simulink library "Radar_Block"  (R2018b)
settings: Solver=VariableStepAuto  StartTime=0.0  StopTime=10.0  RelTol=1e-3
undefined symbols (not defined in the file): ac1dyn_alt0_ft, ac1dyn_lat0_rad, ac1dyn_lon0_rad, uas_rdr_az_bias_rad, uas_rdr_az_random_stddev_rad, uas_rdr_az_tau_s, uas_rdr_debugMode, uas_rdr_dt_s, uas_rdr_el_bias_rad, uas_rdr_el_random_stddev_rad, uas_rdr_el_tau_s, uas_rdr_RCPR_Mode, uas_rdr_RCPR_Range_ft, uas_rdr_reported_errorCovRAE, uas_rdr_rng_bias_ft, uas_rdr_rng_random_stddev_ft, uas_rdr_rng_tau_s, uas_rdr_rngdot_bias_ftps, uas_rdr_rngdot_random_stddev_ftps, uas_rdr_rngdot_tau_s, uas_rdr_seed1, uas_rdr_seed2, uas_rdr_seed3, uas_rdr_seed4, uas_rdr_sns_for_azimuth_deg, uas_rdr_sns_for_elevation_deg
libraries: simulink x7, signalsLib x1, ExtractCovDiag x1
settings Model: Creator=RA24876  LastModifiedBy=BI28030
settings SFSimCC: SimUseLocalCustomCode=off
settings RTWCC: RTWUseLocalCustomCode=off
settings CodeAppCC: StateflowObjectComments=on

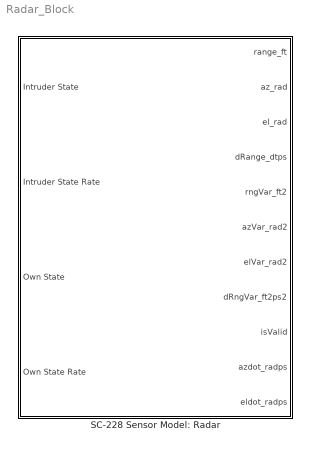
== system Radar_Block ==
  SC-228 Sensor Model: Radar : Subsystem  mask(Tracked Surveillance: Radar){dt_s=uas_rdr_dt_s, lat0_rad=ac1dyn_lat0_rad, lon0_rad=ac1dyn_lon0_rad, alt0_ft=ac1dyn_alt0_ft, sns_for_azimuth_deg=uas_rdr_sns_for_azimuth_deg, sns_for_elevation_deg=uas_rdr_sns_for_elevation_deg, debugMode=uas_rdr_debugMode, rng_random_stddev_ft=uas_rdr_rng_random_stddev_ft, rng_bias_ft=uas_rdr_rng_bias_ft, rng_tau_s=uas_rdr_rng_tau_s, seed1=uas_rdr_seed1, RCPR_Mode=uas_rdr_RCPR_Mode, RCPR_Range_ft=uas_rdr_RCPR_Range_ft, az_random_stddev_rad=uas_rdr_az_random_stddev_rad, az_bias_rad=uas_rdr_az_bias_rad, az_tau_s=uas_rdr_az_tau_s, seed2=uas_rdr_seed2, el_random_stddev_rad=uas_rdr_el_random_stddev_rad, el_bias_rad=uas_rdr_el_bias_rad, el_tau_s=uas_rdr_el_tau_s, seed3=uas_rdr_seed3, rngdot_random_stddev_ftps=uas_rdr_rngdot_random_stddev_ftps, rngdot_bias_ftps=uas_rdr_rngdot_bias_ftps, rngdot_tau_s=uas_rdr_rngdot_tau_s, seed4=uas_rdr_seed4, covRAE=uas_rdr_reported_errorCovRAE}
      mask prompts: dt_s "Timestep"; lat0_rad "ENU Origin Latitude"; lon0_rad "ENU Origin Longitude"; alt0_ft "ENU Origin Altitude"; sns_for_azimuth_deg "Field of Regard: Azimuth Limit (deg)"; sns_for_elevation_deg "Field of Regard: Elevation Limit (deg)"; debugMode "Whether to run in debug mode with inifinite detection range"; rng_random_stddev_ft "Range Random Error Standard Deviation"; rng_bias_ft "Range Bias"; rng_tau_s "Correlation Time"; seed1 "Random Seed"; RCPR_Mode "RCPR Mode (1 = minimum range enabled, 0 = not enabled)"; RCPR_Range_ft "RCPR Range (ft)"; az_random_stddev_rad "Azimuth Random Error Standard Deviation"; az_bias_rad "Azimuth Bias"; az_tau_s "Correlation Time"; seed2 "Random Seed"; el_random_stddev_rad "Elevation Random Error Standard Deviation"; el_bias_rad "Elevation Bias"; el_tau_s "Correlation Time"; seed3 "Random Seed"; rngdot_random_stddev_ftps "Range Rate Random Error Standard Deviation"; rngdot_bias_ftps "Range Rate Bias"; rngdot_tau_s "Correlation Time"; seed4 "Random Seed"; covRAE "Error Covariance"
      mask help: Additive noise model of an on-board radar
      mask Help:
      | Additive noise model of an on-board radar.  Independent noise is added to
      | each of range, azimuth, elevation and their rates.  Noise is colored using
      | weights determined by time constant parameters.
      | 
      | Output takes the form of a AircraftEstimate data bus and a 6x6 error covariance
      | matrix in North-East-Down.  State order in error covariance output is
      | [ posN posE posD velN velE velD ].
      mask DialogControl ParameterTabVar0 Prompt: Tab
      mask DialogControl ParameterTabVar01 Prompt: Range
      mask DialogControl ParameterTabVar012 Prompt: Azimuth
      mask DialogControl ParameterTabVar0123 Prompt: Elevation
      mask DialogControl ParameterTabVar01234 Prompt: Range rate
      mask DialogControl ParameterTabVar01234567 Prompt: Covariance

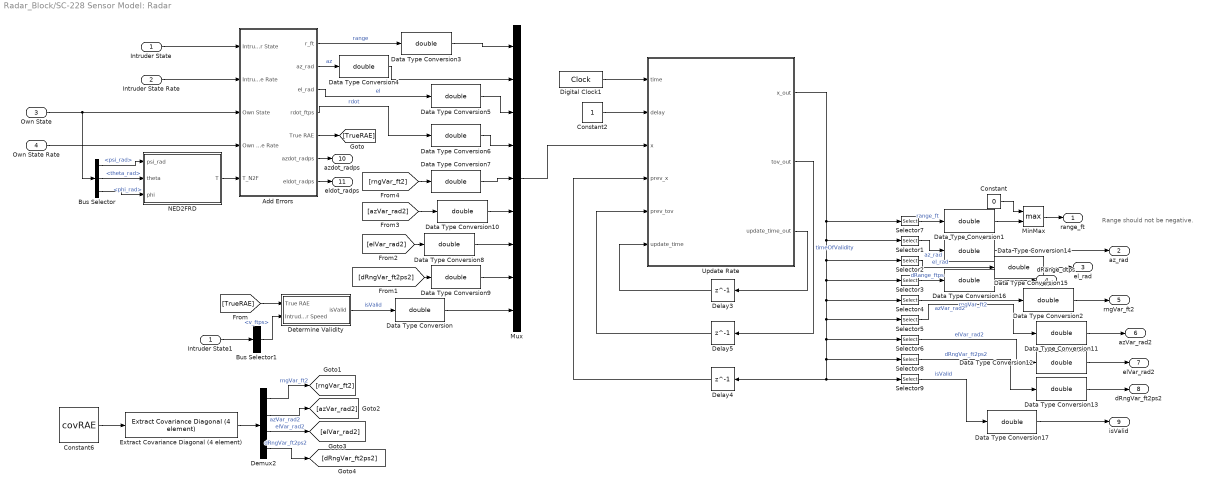
== system Radar_Block/SC-228 Sensor Model: Radar ==
  note: Range should not be negative.
  Intruder State : Inport  OutDataTypeStr=Bus: AircraftState
  Intruder State Rate : Inport  Port=2  OutDataTypeStr=Bus: AircraftStateRate
  Own State : Inport  Port=3  OutDataTypeStr=Bus: AircraftState
  Own State Rate : Inport  Port=4  OutDataTypeStr=Bus: AircraftStateRate
  Add Errors : Subsystem
  Bus Selector : BusSelector  OutputSignals=psi_rad,theta_rad,phi_rad
  Bus Selector1 : BusSelector  OutputSignals=v_ftps
  Constant : Constant  Value=0
  Constant2 : Constant
  Constant6 : Constant  Value=covRAE
  Data Type Conversion{,1..17} (18 alike) : DataTypeConversion  OutDataTypeStr=double
  Delay3 : Delay  DelayLength=1  InitialCondition=1
  Delay4 : Delay  DelayLength=1  InitialCondition=0
  Delay5 : Delay  DelayLength=1  InitialCondition=0
  Demux2 : Demux
  Determine Validity : Subsystem
  Digital Clock1 : DigitalClock  SampleTime=0.1
  Extract Covariance Diagonal (4 element) : ExtractCovDiag/Extract Covariance Diagonal (4 element)  SystemSampleTime=-1
  Intruder State1 : InportShadow  OutDataTypeStr=Bus: AircraftState
  MinMax : MinMax  Function=max  Inputs=2
  Mux : Mux  Inputs=9
  NED2FRD : MATLAB Function  TreatAsAtomicUnit=on
  Selector1 : Selector  InputPortWidth=9  IndexOptions=Index vector (dialog)  Indices=[2]  OutputSizes=1
  Selector2 : Selector  InputPortWidth=9  IndexOptions=Index vector (dialog)  Indices=[3]  OutputSizes=1
  Selector3 : Selector  InputPortWidth=9  IndexOptions=Index vector (dialog)  Indices=[4]  OutputSizes=1
  Selector4 : Selector  InputPortWidth=9  IndexOptions=Index vector (dialog)  Indices=[5]  OutputSizes=1
  Selector5 : Selector  InputPortWidth=9  IndexOptions=Index vector (dialog)  Indices=[6]  OutputSizes=1
  Selector6 : Selector  InputPortWidth=9  IndexOptions=Index vector (dialog)  Indices=[7]  OutputSizes=1
  Selector7 : Selector  InputPortWidth=9  IndexOptions=Index vector (dialog)  Indices=[1]  OutputSizes=1
  Selector8 : Selector  InputPortWidth=9  IndexOptions=Index vector (dialog)  Indices=[8]  OutputSizes=1
  Selector9 : Selector  InputPortWidth=9  IndexOptions=Index vector (dialog)  Indices=[9]  OutputSizes=1
  Update Rate : MATLAB Function  TreatAsAtomicUnit=on
  range_ft : Outport
  az_rad : Outport  Port=2
  el_rad : Outport  Port=3
  dRange_dtps : Outport  Port=4
  rngVar_ft2 : Outport  Port=5
  azVar_rad2 : Outport  Port=6
  elVar_rad2 : Outport  Port=7
  dRngVar_ft2ps2 : Outport  Port=8
  isValid : Outport  Port=9
  azdot_radps : Outport  Port=10
  eldot_radps : Outport  Port=11
  wires:
  Data Type Conversion13/1 -> dRngVar_ft2ps2/1
  Data Type Conversion12/1 -> elVar_rad2/1
  Data Type Conversion11/1 -> azVar_rad2/1
  Data Type Conversion7/1 -> Mux/5
  Data Type Conversion10/1 -> Mux/6
  Data Type Conversion9/1 -> Mux/8
  [dRngVar_ft2ps2] -> Data Type Conversion9/1
  Data Type Conversion8/1 -> Mux/7
  [rngVar_ft2] -> Data Type Conversion7/1
  Data Type Conversion6/1 -> Mux/4
  Data Type Conversion5/1 -> Mux/3
  Data Type Conversion4/1 -> Mux/2
  Data Type Conversion3/1 -> Mux/1
  Data Type Conversion2/1 -> rngVar_ft2/1
  Data Type Conversion1/1 -> MinMax/2
  Add Errors/4(rdot_ftps) -> Data Type Conversion6/1  "rdot"
  Add Errors/3(el_rad) -> Data Type Conversion5/1  "el"
  Add Errors/2(az_rad) -> Data Type Conversion4/1  "az"
  Bus Selector/3 -> NED2FRD/3(phi)  "<phi_rad>"
  Own State/1 -> Bus Selector/1, Add Errors/3(Own State)
  Bus Selector/1 -> NED2FRD/1(psi_rad)  "<psi_rad>"
  Bus Selector/2 -> NED2FRD/2(theta)  "<theta_rad>"
  Intruder State/1 -> Add Errors/1(Intruder State)
  Add Errors/1(r_ft) -> Data Type Conversion3/1  "range"
  NED2FRD/1(T) -> Add Errors/5(T_N2F)
  Intruder State Rate/1 -> Add Errors/2(Intruder State Rate)
  Own State Rate/1 -> Add Errors/4(Own State Rate)
  Add Errors/5(True RAE) -> [TrueRAE]
  [TrueRAE] -> Determine Validity/1(True RAE)
  Determine Validity/1(isValid) -> Data Type Conversion/1  "isValid"
  Digital Clock1/1 -> Update Rate/1(time)
  Constant2/1 -> Update Rate/2(delay)
  [azVar_rad2] -> Data Type Conversion10/1
  [elVar_rad2] -> Data Type Conversion8/1
  Mux/1 -> Update Rate/3(x)
  Delay5/1 -> Update Rate/5(prev_tov)
  Update Rate/2(tov_out) -> Delay5/1  "timeOfValidity"
  Delay3/1 -> Update Rate/6(update_time)
  Delay4/1 -> Update Rate/4(prev_x)
  Update Rate/3(update_time_out) -> Delay3/1
  Update Rate/1(x_out) -> Selector2/1, Selector3/1, Selector4/1, Selector5/1, Selector6/1, Selector8/1, Selector9/1, Delay4/1, Selector1/1, Selector7/1
  Selector7/1 -> Data Type Conversion1/1  "range_ft"
  Selector1/1 -> Data Type Conversion14/1  "az_rad"
  Selector2/1 -> Data Type Conversion15/1  "el_rad"
  Selector3/1 -> Data Type Conversion16/1  "dRange_ftps"
  Selector4/1 -> Data Type Conversion2/1  "rngVar_ft2"
  Selector5/1 -> Data Type Conversion11/1  "azVar_rad2"
  Selector6/1 -> Data Type Conversion12/1  "elVar_rad2"
  Selector8/1 -> Data Type Conversion13/1  "dRngVar_ft2ps2"
  Selector9/1 -> Data Type Conversion17/1  "isValid"
  Intruder State1/1 -> Bus Selector1/1
  Bus Selector1/1 -> Determine Validity/2(Intruder Speed)  "<v_ftps>"
  Constant6/1 -> Extract Covariance Diagonal (4 element)/1
  Extract Covariance Diagonal (4 element)/1 -> Demux2/1
  Demux2/1 -> [rngVar_ft2]  "rngVar_ft2"
  Demux2/2 -> [azVar_rad2]  "azVar_rad2"
  Demux2/3 -> [elVar_rad2]  "elVar_rad2"
  Demux2/4 -> [dRngVar_ft2ps2]  "dRngVar_ft2ps2"
  Data Type Conversion/1 -> Mux/9
  MinMax/1 -> range_ft/1
  Constant/1 -> MinMax/1
  Data Type Conversion14/1 -> az_rad/1
  Data Type Conversion15/1 -> el_rad/1
  Data Type Conversion16/1 -> dRange_dtps/1
  Data Type Conversion17/1 -> isValid/1
  Add Errors/6(azdot_radps) -> azdot_radps/1
  Add Errors/7(eldot_radps) -> eldot_radps/1

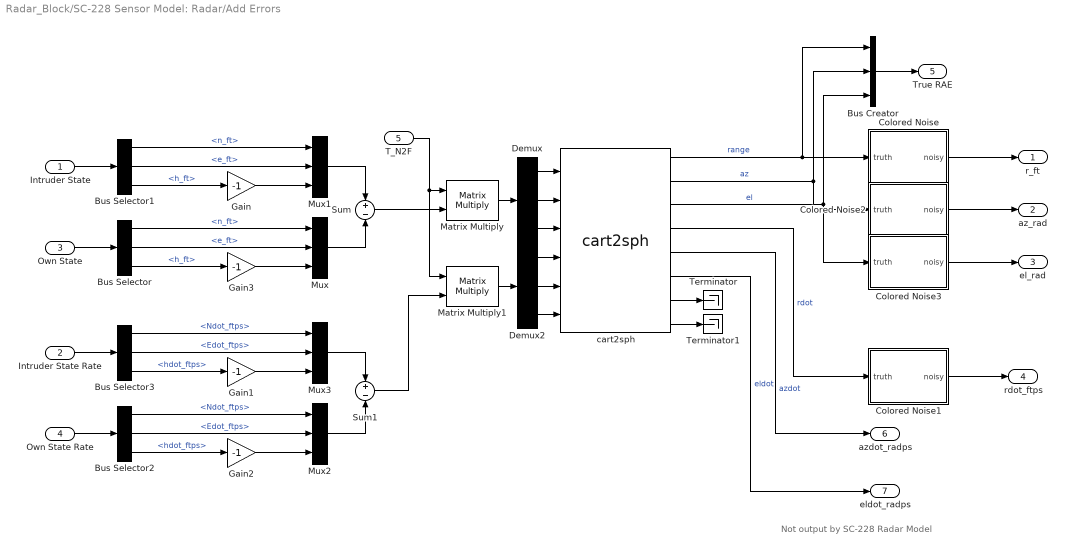
== system Radar_Block/SC-228 Sensor Model: Radar/Add Errors ==
  note: Not output by SC-228 Radar Model
  Intruder State : Inport  OutDataTypeStr=Bus: AircraftState
  Intruder State Rate : Inport  Port=2  OutDataTypeStr=Bus: AircraftStateRate
  Own State : Inport  Port=3  OutDataTypeStr=Bus: AircraftState
  Own State Rate : Inport  Port=4  OutDataTypeStr=Bus: AircraftStateRate
  T_N2F : Inport  Port=5
  Bus Creator : BusCreator  Inputs=3
  Bus Selector : BusSelector  OutputSignals=n_ft,e_ft,h_ft
  Bus Selector1 : BusSelector  OutputSignals=n_ft,e_ft,h_ft
  Bus Selector2 : BusSelector  OutputSignals=Ndot_ftps,Edot_ftps,hdot_ftps
  Bus Selector3 : BusSelector  OutputSignals=Ndot_ftps,Edot_ftps,hdot_ftps
  Colored Noise : Subsystem  mask(Colored Noise){sig=rng_random_stddev_ft, bias=rng_bias_ft, tau=rng_tau_s, dt=dt_s, seed=seed1}
      mask prompts: sig "Random error standard deviation"; bias "Bias error"; tau "Correlation time"; dt "Track update time"; seed "Random Seed"
      mask help: Generates a noisy state variable estimate using the ABSAA colored noise model. Set correlation time to zero for white noise.
      mask Help:
      | Generates a noisy state variable estimate using the AF Common ABSAA error
      | model.  Time correlation of the error is defined by an exponential decay
      | of K = exp(-tau/dt), where tau is the correlation time and dt is the time
      | between track updates.  The track error at time t is then:
      | 
      |     err(t) = K*err(t-1) + N(0,(1-K^2)*sig^2) + bias
      | 
      | where N(x,y) is a Gaussian noise process with mean x and variance y and
      | with random number generator seeded with the integer 'seed'.
      | 
      | The random noise process must be initialized with an error drawn from
      | N(0,sig^2).
      | 
      | The noise model can be used to produce white noise by setting tau to zero.
  Colored Noise1 : Subsystem  mask(Colored Noise){sig=rngdot_random_stddev_ftps, bias=rngdot_bias_ftps, tau=rngdot_tau_s, dt=dt_s, seed=seed4}
      mask prompts: sig "Random error standard deviation"; bias "Bias error"; tau "Correlation time"; dt "Track update time"; seed "Random Seed"
      mask help: Generates a noisy state variable estimate using the ABSAA colored noise model. Set correlation time to zero for white noise.
      mask Help:
      | Generates a noisy state variable estimate using the AF Common ABSAA error
      | model.  Time correlation of the error is defined by an exponential decay
      | of K = exp(-tau/dt), where tau is the correlation time and dt is the time
      | between track updates.  The track error at time t is then:
      | 
      |     err(t) = K*err(t-1) + N(0,(1-K^2)*sig^2) + bias
      | 
      | where N(x,y) is a Gaussian noise process with mean x and variance y and
      | with random number generator seeded with the integer 'seed'.
      | 
      | The random noise process must be initialized with an error drawn from
      | N(0,sig^2).
      | 
      | The noise model can be used to produce white noise by setting tau to zero.
  Colored Noise2 : Subsystem  mask(Colored Noise){sig=az_random_stddev_rad, bias=az_bias_rad, tau=az_tau_s, dt=dt_s, seed=seed2}
      mask prompts: sig "Random error standard deviation"; bias "Bias error"; tau "Correlation time"; dt "Track update time"; seed "Random Seed"
      mask help: Generates a noisy state variable estimate using the ABSAA colored noise model. Set correlation time to zero for white noise.
      mask Help:
      | Generates a noisy state variable estimate using the AF Common ABSAA error
      | model.  Time correlation of the error is defined by an exponential decay
      | of K = exp(-tau/dt), where tau is the correlation time and dt is the time
      | between track updates.  The track error at time t is then:
      | 
      |     err(t) = K*err(t-1) + N(0,(1-K^2)*sig^2) + bias
      | 
      | where N(x,y) is a Gaussian noise process with mean x and variance y and
      | with random number generator seeded with the integer 'seed'.
      | 
      | The random noise process must be initialized with an error drawn from
      | N(0,sig^2).
      | 
      | The noise model can be used to produce white noise by setting tau to zero.
  Colored Noise3 : Subsystem  mask(Colored Noise){sig=el_random_stddev_rad, bias=el_bias_rad, tau=el_tau_s, dt=dt_s, seed=seed3}
      mask prompts: sig "Random error standard deviation"; bias "Bias error"; tau "Correlation time"; dt "Track update time"; seed "Random Seed"
      mask help: Generates a noisy state variable estimate using the ABSAA colored noise model. Set correlation time to zero for white noise.
      mask Help:
      | Generates a noisy state variable estimate using the AF Common ABSAA error
      | model.  Time correlation of the error is defined by an exponential decay
      | of K = exp(-tau/dt), where tau is the correlation time and dt is the time
      | between track updates.  The track error at time t is then:
      | 
      |     err(t) = K*err(t-1) + N(0,(1-K^2)*sig^2) + bias
      | 
      | where N(x,y) is a Gaussian noise process with mean x and variance y and
      | with random number generator seeded with the integer 'seed'.
      | 
      | The random noise process must be initialized with an error drawn from
      | N(0,sig^2).
      | 
      | The noise model can be used to produce white noise by setting tau to zero.
  Demux : Demux  Outputs=3
  Demux2 : Demux  Outputs=3
  Gain{,1..3} (4 alike) : Gain  Gain=-1
  Matrix Multiply : Product  Multiplication=Matrix(*)
  Matrix Multiply1 : Product  Multiplication=Matrix(*)
  Mux{,1..3} (4 alike) : Mux  Inputs=3
  Sum : Sum  Inputs=+-
  Sum1 : Sum  Inputs=+-
  Terminator : Terminator
  Terminator1 : Terminator
  cart2sph : signalsLib/Signals/Coordinate Transformations/cart2sph
      settings: SourceProductName=DEGASv1: Signals Library
  r_ft : Outport
  az_rad : Outport  Port=2
  el_rad : Outport  Port=3
  rdot_ftps : Outport  Port=4
  True RAE : Outport  Port=5
  azdot_radps : Outport  Port=6
  eldot_radps : Outport  Port=7
  wires:
  cart2sph/8 -> Terminator1/1
  cart2sph/7 -> Terminator/1
  Demux2/3 -> cart2sph/6
  Demux2/2 -> cart2sph/5
  Demux2/1 -> cart2sph/4
  cart2sph/4 -> Colored Noise1/1(truth)  "rdot"
  Matrix Multiply1/1 -> Demux2/1
  Demux/1 -> cart2sph/1
  Demux/2 -> cart2sph/2
  Demux/3 -> cart2sph/3
  Matrix Multiply/1 -> Demux/1
  Sum1/1 -> Matrix Multiply1/2
  Sum/1 -> Matrix Multiply/2
  T_N2F/1 -> Matrix Multiply/1, Matrix Multiply1/1
  Gain3/1 -> Mux/3
  Gain/1 -> Mux1/3
  Gain2/1 -> Mux2/3
  Gain1/1 -> Mux3/3
  Mux2/1 -> Sum1/2
  Mux3/1 -> Sum1/1
  Bus Selector2/2 -> Mux2/2  "<Edot_ftps>"
  Bus Selector2/1 -> Mux2/1  "<Ndot_ftps>"
  Bus Selector2/3 -> Gain2/1  "<hdot_ftps>"
  Own State Rate/1 -> Bus Selector2/1
  Intruder State Rate/1 -> Bus Selector3/1
  Bus Selector3/2 -> Mux3/2  "<Edot_ftps>"
  Bus Selector3/1 -> Mux3/1  "<Ndot_ftps>"
  Bus Selector3/3 -> Gain1/1  "<hdot_ftps>"
  Mux/1 -> Sum/2
  Mux1/1 -> Sum/1
  Intruder State/1 -> Bus Selector1/1
  Bus Selector1/2 -> Mux1/2  "<e_ft>"
  Bus Selector1/1 -> Mux1/1  "<n_ft>"
  Bus Selector1/3 -> Gain/1  "<h_ft>"
  Bus Selector/2 -> Mux/2  "<e_ft>"
  Bus Selector/1 -> Mux/1  "<n_ft>"
  Bus Selector/3 -> Gain3/1  "<h_ft>"
  Own State/1 -> Bus Selector/1
  cart2sph/1 -> Colored Noise/1(truth), Bus Creator/1  "range"
  cart2sph/2 -> Bus Creator/2, Colored Noise2/1(truth)  "az"
  cart2sph/3 -> Bus Creator/3, Colored Noise3/1(truth)  "el"
  cart2sph/5 -> azdot_radps/1  "azdot"
  cart2sph/6 -> eldot_radps/1  "eldot"
  Colored Noise/1(noisy) -> r_ft/1
  Colored Noise1/1(noisy) -> rdot_ftps/1
  Colored Noise2/1(noisy) -> az_rad/1
  Colored Noise3/1(noisy) -> el_rad/1
  Bus Creator/1 -> True RAE/1

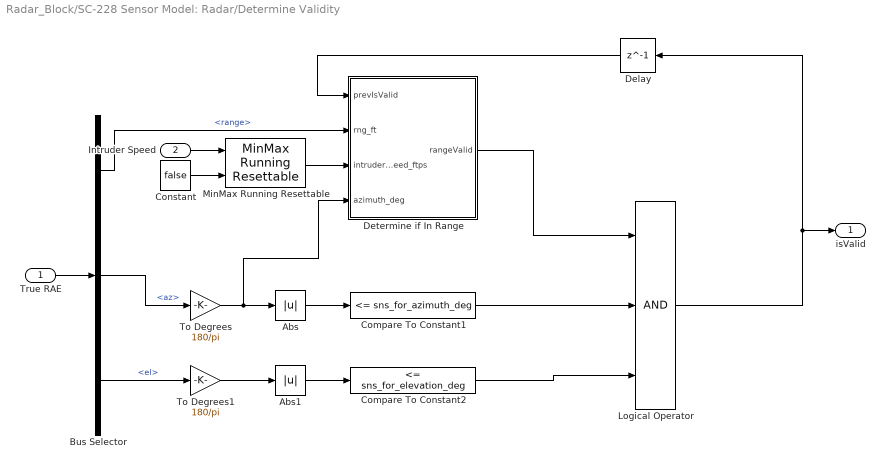
== system Radar_Block/SC-228 Sensor Model: Radar/Determine Validity ==
  True RAE : Inport
  Intruder Speed : Inport  Port=2
  Abs : Abs
  Abs1 : Abs
  Bus Selector : BusSelector  OutputSignals=range,az,el
  Compare To Constant1 : simulink/Logic and Bit Operations/Compare To Constant  relop=<=  const=sns_for_azimuth_deg  OutDataTypeStr=boolean
  Compare To Constant2 : simulink/Logic and Bit Operations/Compare To Constant  relop=<=  const=sns_for_elevation_deg  OutDataTypeStr=boolean
  Constant : Constant  Value=false
  Delay : Delay  DelayLength=1  InitialCondition=0
  Determine if In Range : Subsystem  mask{debugMode=debugMode}
      mask prompts: debugMode "Whether to run in Debug Mode with infinite detection range"
  Logical Operator : Logic  Inputs=3  AllPortsSameDT=off  OutDataTypeStr=boolean
  MinMax Running Resettable : simulink/Math Operations/MinMax Running Resettable  Function=max  vinit=0.0
  To Degrees : Gain  Gain=180/pi
  To Degrees1 : Gain  Gain=180/pi
  isValid : Outport
  wires:
  True RAE/1 -> Bus Selector/1
  Logical Operator/1 -> isValid/1, Delay/1
  Abs/1 -> Compare To Constant1/1
  Bus Selector/2 -> To Degrees/1  "<az>"
  Bus Selector/3 -> To Degrees1/1  "<el>"
  Abs1/1 -> Compare To Constant2/1
  Compare To Constant1/1 -> Logical Operator/2
  Compare To Constant2/1 -> Logical Operator/3
  To Degrees1/1 -> Abs1/1
  Bus Selector/1 -> Determine if In Range/2(rng_ft)  "<range>"
  Determine if In Range/1(rangeValid) -> Logical Operator/1
  Intruder Speed/1 -> MinMax Running Resettable/1
  Constant/1 -> MinMax Running Resettable/2
  MinMax Running Resettable/1 -> Determine if In Range/3(intruderSpeed_ftps)
  To Degrees/1 -> Determine if In Range/4(azimuth_deg), Abs/1
  Delay/1 -> Determine if In Range/1(prevIsValid)

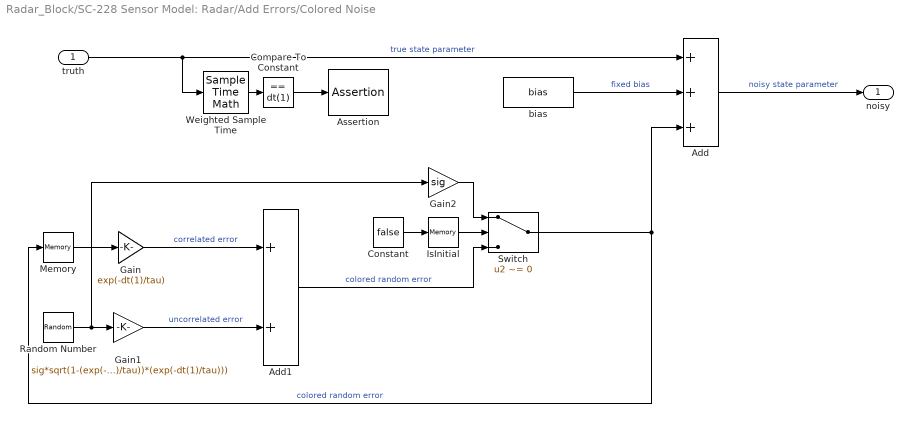
== system Radar_Block/SC-228 Sensor Model: Radar/Add Errors/Colored Noise ==
  truth : Inport
  Add : Sum  Inputs=+++  SampleTime=dt
  Add1 : Sum  SampleTime=dt
  Assertion : Assertion
  Compare To Constant : simulink/Logic and Bit Operations/Compare To Constant  relop===  const=dt(1)  OutDataTypeStr=boolean
  Constant : Constant  Value=false
  Gain : Gain  Gain=exp(-dt(1)/tau)  SampleTime=dt
  Gain1 : Gain  Gain=sig*sqrt(1-(exp(-dt(1)/tau))*(exp(-dt(1)/tau)))
  Gain2 : Gain  Gain=sig
  IsInitial : Memory  InitialCondition=true  InheritSampleTime=on
  Memory : Memory  InheritSampleTime=on
  Random Number : RandomNumber  Seed=seed  SampleTime=dt_s
  Switch : Switch  Criteria=u2 ~= 0  SampleTime=dt
  Weighted Sample Time : SampleTimeMath  TsampMathOp=Ts Only
  bias : Constant  Value=bias
  noisy : Outport
  wires:
  Gain1/1 -> Add1/2  "uncorrelated error"
  Switch/1 -> Memory/1, Add/3  "colored random error"
  bias/1 -> Add/2  "fixed bias"
  Random Number/1 -> Gain2/1, Gain1/1
  Gain/1 -> Add1/1  "correlated error"
  Add/1 -> noisy/1  "noisy state parameter"
  truth/1 -> Weighted Sample Time/1, Add/1  "true state parameter"
  Memory/1 -> Gain/1
  Constant/1 -> IsInitial/1
  IsInitial/1 -> Switch/2
  Add1/1 -> Switch/3  "colored random error"
  Gain2/1 -> Switch/1
  Weighted Sample Time/1 -> Compare To Constant/1
  Compare To Constant/1 -> Assertion/1

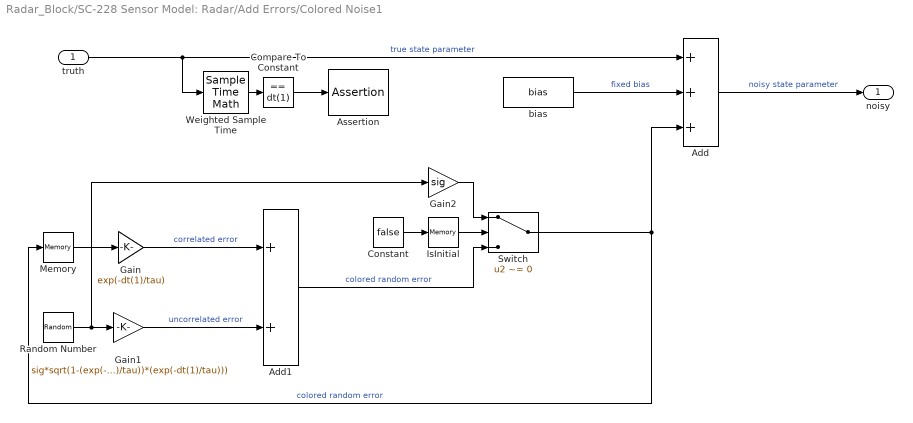
== system Radar_Block/SC-228 Sensor Model: Radar/Add Errors/Colored Noise1 ==
  truth : Inport
  Add : Sum  Inputs=+++  SampleTime=dt
  Add1 : Sum  SampleTime=dt
  Assertion : Assertion
  Compare To Constant : simulink/Logic and Bit Operations/Compare To Constant  relop===  const=dt(1)  OutDataTypeStr=boolean
  Constant : Constant  Value=false
  Gain : Gain  Gain=exp(-dt(1)/tau)  SampleTime=dt
  Gain1 : Gain  Gain=sig*sqrt(1-(exp(-dt(1)/tau))*(exp(-dt(1)/tau)))
  Gain2 : Gain  Gain=sig
  IsInitial : Memory  InitialCondition=true  InheritSampleTime=on
  Memory : Memory  InheritSampleTime=on
  Random Number : RandomNumber  Seed=seed  SampleTime=dt_s
  Switch : Switch  Criteria=u2 ~= 0  SampleTime=dt
  Weighted Sample Time : SampleTimeMath  TsampMathOp=Ts Only
  bias : Constant  Value=bias
  noisy : Outport
  wires:
  Gain1/1 -> Add1/2  "uncorrelated error"
  Switch/1 -> Memory/1, Add/3  "colored random error"
  bias/1 -> Add/2  "fixed bias"
  Random Number/1 -> Gain2/1, Gain1/1
  Gain/1 -> Add1/1  "correlated error"
  Add/1 -> noisy/1  "noisy state parameter"
  truth/1 -> Weighted Sample Time/1, Add/1  "true state parameter"
  Memory/1 -> Gain/1
  Constant/1 -> IsInitial/1
  IsInitial/1 -> Switch/2
  Add1/1 -> Switch/3  "colored random error"
  Gain2/1 -> Switch/1
  Weighted Sample Time/1 -> Compare To Constant/1
  Compare To Constant/1 -> Assertion/1

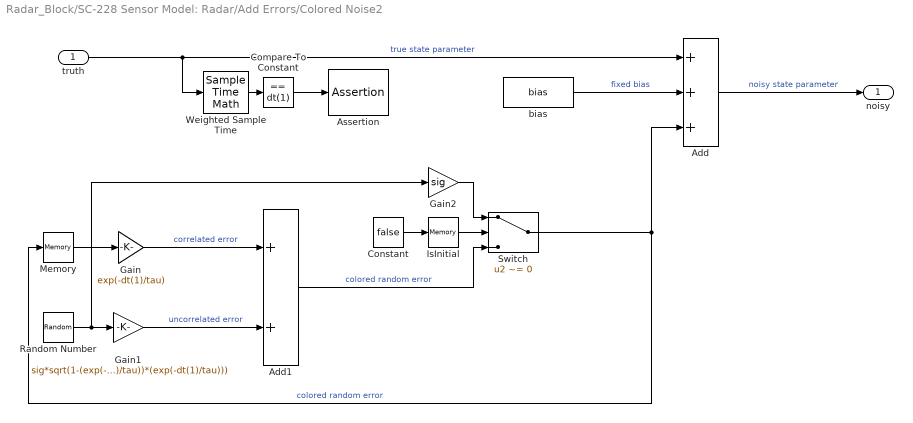
== system Radar_Block/SC-228 Sensor Model: Radar/Add Errors/Colored Noise2 ==
  truth : Inport
  Add : Sum  Inputs=+++  SampleTime=dt
  Add1 : Sum  SampleTime=dt
  Assertion : Assertion
  Compare To Constant : simulink/Logic and Bit Operations/Compare To Constant  relop===  const=dt(1)  OutDataTypeStr=boolean
  Constant : Constant  Value=false
  Gain : Gain  Gain=exp(-dt(1)/tau)  SampleTime=dt
  Gain1 : Gain  Gain=sig*sqrt(1-(exp(-dt(1)/tau))*(exp(-dt(1)/tau)))
  Gain2 : Gain  Gain=sig
  IsInitial : Memory  InitialCondition=true  InheritSampleTime=on
  Memory : Memory  InheritSampleTime=on
  Random Number : RandomNumber  Seed=seed  SampleTime=dt_s
  Switch : Switch  Criteria=u2 ~= 0  SampleTime=dt
  Weighted Sample Time : SampleTimeMath  TsampMathOp=Ts Only
  bias : Constant  Value=bias
  noisy : Outport
  wires:
  Gain1/1 -> Add1/2  "uncorrelated error"
  Switch/1 -> Memory/1, Add/3  "colored random error"
  bias/1 -> Add/2  "fixed bias"
  Random Number/1 -> Gain2/1, Gain1/1
  Gain/1 -> Add1/1  "correlated error"
  Add/1 -> noisy/1  "noisy state parameter"
  truth/1 -> Weighted Sample Time/1, Add/1  "true state parameter"
  Memory/1 -> Gain/1
  Constant/1 -> IsInitial/1
  IsInitial/1 -> Switch/2
  Add1/1 -> Switch/3  "colored random error"
  Gain2/1 -> Switch/1
  Weighted Sample Time/1 -> Compare To Constant/1
  Compare To Constant/1 -> Assertion/1

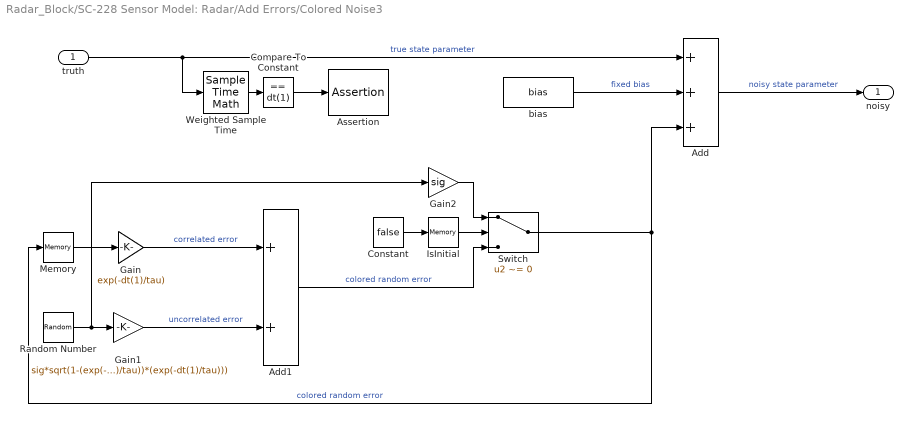
== system Radar_Block/SC-228 Sensor Model: Radar/Add Errors/Colored Noise3 ==
  truth : Inport
  Add : Sum  Inputs=+++  SampleTime=dt
  Add1 : Sum  SampleTime=dt
  Assertion : Assertion
  Compare To Constant : simulink/Logic and Bit Operations/Compare To Constant  relop===  const=dt(1)  OutDataTypeStr=boolean
  Constant : Constant  Value=false
  Gain : Gain  Gain=exp(-dt(1)/tau)  SampleTime=dt
  Gain1 : Gain  Gain=sig*sqrt(1-(exp(-dt(1)/tau))*(exp(-dt(1)/tau)))
  Gain2 : Gain  Gain=sig
  IsInitial : Memory  InitialCondition=true  InheritSampleTime=on
  Memory : Memory  InheritSampleTime=on
  Random Number : RandomNumber  Seed=seed  SampleTime=dt_s
  Switch : Switch  Criteria=u2 ~= 0  SampleTime=dt
  Weighted Sample Time : SampleTimeMath  TsampMathOp=Ts Only
  bias : Constant  Value=bias
  noisy : Outport
  wires:
  Gain1/1 -> Add1/2  "uncorrelated error"
  Switch/1 -> Memory/1, Add/3  "colored random error"
  bias/1 -> Add/2  "fixed bias"
  Random Number/1 -> Gain2/1, Gain1/1
  Gain/1 -> Add1/1  "correlated error"
  Add/1 -> noisy/1  "noisy state parameter"
  truth/1 -> Weighted Sample Time/1, Add/1  "true state parameter"
  Memory/1 -> Gain/1
  Constant/1 -> IsInitial/1
  IsInitial/1 -> Switch/2
  Add1/1 -> Switch/3  "colored random error"
  Gain2/1 -> Switch/1
  Weighted Sample Time/1 -> Compare To Constant/1
  Compare To Constant/1 -> Assertion/1

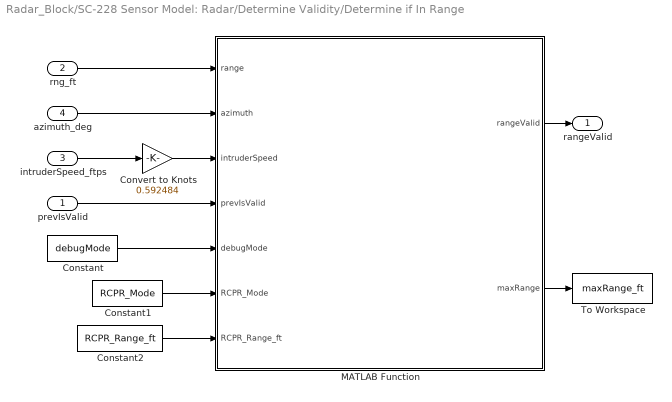
== system Radar_Block/SC-228 Sensor Model: Radar/Determine Validity/Determine if In Range ==
  prevIsValid : Inport
  rng_ft : Inport  Port=2
  intruderSpeed_ftps : Inport  Port=3
  azimuth_deg : Inport  Port=4
  Constant : Constant  Value=debugMode
  Constant1 : Constant  Value=RCPR_Mode
  Constant2 : Constant  Value=RCPR_Range_ft
  Convert to Knots : Gain  Gain=0.592484
  MATLAB Function : MATLAB Function  TreatAsAtomicUnit=on
  To Workspace : ToWorkspace  VariableName=maxRange_ft  SaveFormat=Timeseries  SampleTime=-1
  rangeValid : Outport
  wires:
  Constant2/1 -> MATLAB Function/7(RCPR_Range_ft)
  Constant1/1 -> MATLAB Function/6(RCPR_Mode)
  rng_ft/1 -> MATLAB Function/1(range)
  MATLAB Function/1(rangeValid) -> rangeValid/1
  intruderSpeed_ftps/1 -> Convert to Knots/1
  prevIsValid/1 -> MATLAB Function/4(prevIsValid)
  Convert to Knots/1 -> MATLAB Function/3(intruderSpeed)
  azimuth_deg/1 -> MATLAB Function/2(azimuth)
  Constant/1 -> MATLAB Function/5(debugMode)
  MATLAB Function/2(maxRange) -> To Workspace/1

== matlab function Radar_Block/SC-228 Sensor Model: Radar/Determine Validity/Determine if In Range/MATLAB Function ==
  data: range input; azimuth input; intruderSpeed input; rangeValid output; prevIsValid input; debugMode input; maxRange output; RCPR_Mode input; RCPR_Range_ft input
function [rangeValid, maxRange] = determineRangeValidity(range, azimuth, intruderSpeed, prevIsValid, debugMode, RCPR_Mode, RCPR_Range_ft)
%#codegen
maxRange = 0;

if(debugMode)
    if(RCPR_Mode)
        rangeValid = range >= RCPR_Range_ft;
    else
        rangeValid = true; 
    end
    maxRange = Inf;
    return;
end

azimuth = abs(azimuth);

if(intruderSpeed<100)
    DR = 5.4*6070;
    %Do not perform scale factor correction once track is established
    %DR scale factor is linearly interpolated between levels
    if(azimuth<=30)
        maxRange = DR*(1-0.33*(azimuth-0)/(30-0)*~prevIsValid);
    elseif(azimuth<=60)
        maxRange = DR*(1-(0.33+0.22*(azimuth-30)/(60-30))*~prevIsValid);   
    elseif(azimuth<=90)
        maxRange = DR*(1-(0.55+0.1*(azimuth-60)/(90-60))*~prevIsValid);   
    elseif(azimuth<=110)
        maxRange = DR*(1-(0.65+0.0*(azimuth-90)/(110-90))*~prevIsValid);   
    end
    
elseif (intruderSpeed>=100 && intruderSpeed<=130)
    DR = 6.0*6070;
    %Do not perform scale factor correction once track is established
    %DR scale factor is linearly interpolated between levels
    if(azimuth<=30)
        maxRange = DR*(1-0.22*(azimuth-0)/(30-0)*~prevIsValid);
    elseif(azimuth<=60)
        maxRange = DR*(1-(0.22+0.26*(azimuth-30)/(60-30))*~prevIsValid);   
    elseif(azimuth<=90)
        maxRange = DR*(1-(0.48+0.09*(azimuth-60)/(90-60))*~prevIsValid);   
    elseif(azimuth<=110)
        maxRange = DR*(1-(0.57+0.0*(azimuth-90)/(110-90))*~prevIsValid);   
    end
    
elseif(intruderSpeed>130)
    DR = 6.7*6070;
    %Do not perform scale factor correction once track is established
    %DR scale factor is linearly interpolated between levels
    if(azimuth<=30)
        maxRange = DR*(1-0.16*(azimuth-0)/(30-0)*~prevIsValid);
    elseif(azimuth<=60)
        maxRange = DR*(1-(0.16+0.24*(azimuth-30)/(60-30))*~prevIsValid);   
    elseif(azimuth<=90)
        maxRange = DR*(1-(0.4+0.05*(azimuth-60)/(90-60))*~prevIsValid);   
    elseif(azimuth<=110)
        maxRange = DR*(1-(0.45+0.0*(azimuth-90)/(110-90))*~prevIsValid);   
    end
    
end
    
if(RCPR_Mode)
   rangeValid = range <= maxRange & range >= RCPR_Range_ft;  
else
   rangeValid = range <= maxRange;  
end

== matlab function Radar_Block/SC-228 Sensor Model: Radar/NED2FRD ==
  data: psi_rad input; T output; theta input; phi input
function T = Transform_NED2FRD(psi_rad,theta,phi)
%#codegen

yaw = [ cos(psi_rad) sin(psi_rad) 0;
       -sin(psi_rad) cos(psi_rad) 0;
               0        0 1 ];
           
pitch = [ cos(theta) 0 -sin(theta);
                   0 1           0;
          sin(theta) 0  cos(theta) ];
      
roll = [ 1         0        0;
         0  cos(phi) sin(phi);
         0 -sin(phi) cos(phi) ];
     
T = roll*pitch*yaw;     % transformation FROM geographic coord TO body coord

== matlab function Radar_Block/SC-228 Sensor Model: Radar/Update Rate ==
  data: time input; x_out output; tov_out output; delay input; x input; prev_x input; prev_tov input; update_time input; update_time_out output
function [x_out,tov_out,update_time_out] = fcn(time,delay,x,prev_x,prev_tov,update_time)
%#codegen

if time-update_time>=-0.001 % pass out new output
    update_time_out = time+delay; 
    x_out = x;
    tov_out = time;
else % continue passing out old output
    x_out = prev_x; 
    update_time_out = update_time;
    tov_out = prev_tov;
end
